simulink model "Grid_Forming_Converters_Microgrid_Github"  (R2020b)
settings: Solver=VariableStepAuto  StartTime=0.0  StopTime=1  RelTol=1e-3
values from neighbouring files (symbols this model uses):
  C_fi_1DG = 50*10^-6    (= 5e-05)    [Script_Primary_Secondary_Controller_GITHUB.m]
  C_fi_2DG = 50*10^-6    (= 5e-05)    [Script_Primary_Secondary_Controller_GITHUB.m]
  C_fi_3DG = 50*10^-6    (= 5e-05)    [Script_Primary_Secondary_Controller_GITHUB.m]
  C_fi_4DG = 50*10^-6    (= 5e-05)    [Script_Primary_Secondary_Controller_GITHUB.m]
  Kff_i_1DG = 0.75    [Script_Primary_Secondary_Controller_GITHUB.m]
  Kff_i_2DG = 0.75    [Script_Primary_Secondary_Controller_GITHUB.m]
  Kff_i_3DG = 0.75    [Script_Primary_Secondary_Controller_GITHUB.m]
  Kff_i_4DG = 0.75    [Script_Primary_Secondary_Controller_GITHUB.m]
  ki = 142500    [Script_Primary_Secondary_Controller_GITHUB.m]
  Kii_1DG = 20000    [Script_Primary_Secondary_Controller_GITHUB.m]
  Kii_2DG = 20000    [Script_Primary_Secondary_Controller_GITHUB.m]
  Kii_3DG = 16000    [Script_Primary_Secondary_Controller_GITHUB.m]
  Kii_4DG = 16000    [Script_Primary_Secondary_Controller_GITHUB.m]
  Kiv_1DG = 420    [Script_Primary_Secondary_Controller_GITHUB.m]
  Kiv_2DG = 420    [Script_Primary_Secondary_Controller_GITHUB.m]
  Kiv_3DG = 390    [Script_Primary_Secondary_Controller_GITHUB.m]
  Kiv_4DG = 390    [Script_Primary_Secondary_Controller_GITHUB.m]
  kp = 285    [Script_Primary_Secondary_Controller_GITHUB.m]
  Kpi_1DG = 15    [Script_Primary_Secondary_Controller_GITHUB.m]
  Kpi_2DG = 15    [Script_Primary_Secondary_Controller_GITHUB.m]
  Kpi_3DG = 10.5    [Script_Primary_Secondary_Controller_GITHUB.m]
  Kpi_4DG = 10.5    [Script_Primary_Secondary_Controller_GITHUB.m]
  Kpv_1DG = 0.1    [Script_Primary_Secondary_Controller_GITHUB.m]
  Kpv_2DG = 0.1    [Script_Primary_Secondary_Controller_GITHUB.m]
  Kpv_3DG = 0.05    [Script_Primary_Secondary_Controller_GITHUB.m]
  Kpv_4DG = 0.05    [Script_Primary_Secondary_Controller_GITHUB.m]
  L_ci_1DG = 0.35*10^-3    (= 0.00035)    [Script_Primary_Secondary_Controller_GITHUB.m]
  L_ci_2DG = 0.35*10^-3    (= 0.00035)    [Script_Primary_Secondary_Controller_GITHUB.m]
  L_fi_1DG = 1.35*10^-3    (= 0.00135)    [Script_Primary_Secondary_Controller_GITHUB.m]
  L_fi_2DG = 1.35*10^-3    (= 0.00135)    [Script_Primary_Secondary_Controller_GITHUB.m]
  L_fi_3DG = 1.35*10^-3    (= 0.00135)    [Script_Primary_Secondary_Controller_GITHUB.m]
  L_fi_4DG = 1.35*10^-3    (= 0.00135)    [Script_Primary_Secondary_Controller_GITHUB.m]
  L_line_1 = 318*10^-6    (= 0.000318)    [Script_Primary_Secondary_Controller_GITHUB.m]
  L_line_2 = 1847*10^-6    (= 0.001847)    [Script_Primary_Secondary_Controller_GITHUB.m]
  L_line_3 = 318*10^-6    (= 0.000318)    [Script_Primary_Secondary_Controller_GITHUB.m]
  L_load_1 = (X_load_1)/(2*pi*f)    (= 0.0477464829276)    [Script_Primary_Secondary_Controller_GITHUB.m]
  L_load_2 = (X_load_2)/(2*pi*f)    (= 0.0318309886184)    [Script_Primary_Secondary_Controller_GITHUB.m]
  L_load_3 = (X_load_3)/(2*pi*f)    (= 0.0318309886184)    [Script_Primary_Secondary_Controller_GITHUB.m]
  L_load_4 = (X_load_4)/(2*pi*f)    (= 0.0477464829276)    [Script_Primary_Secondary_Controller_GITHUB.m]
  m_P_1DG = 9.4*10^-5    (= 9.4e-05)    [Script_Primary_Secondary_Controller_GITHUB.m]
  m_P_2DG = 9.4*10^-5    (= 9.4e-05)    [Script_Primary_Secondary_Controller_GITHUB.m]
  m_P_3DG = 12.5*10^-5    (= 0.000125)    [Script_Primary_Secondary_Controller_GITHUB.m]
  m_P_4DG = 12.5*10^-5    (= 0.000125)    [Script_Primary_Secondary_Controller_GITHUB.m]
  n_Q_1DG = 1.3*10^-3    (= 0.0013)    [Script_Primary_Secondary_Controller_GITHUB.m]
  n_Q_2DG = 1.3*10^-3    (= 0.0013)    [Script_Primary_Secondary_Controller_GITHUB.m]
  n_Q_3DG = 1.5*10^-3    (= 0.0015)    [Script_Primary_Secondary_Controller_GITHUB.m]
  n_Q_4DG = 1.5*10^-3    (= 0.0015)    [Script_Primary_Secondary_Controller_GITHUB.m]
  R_ci_1DG = 0.03    [Script_Primary_Secondary_Controller_GITHUB.m]
  R_ci_2DG = 0.03    [Script_Primary_Secondary_Controller_GITHUB.m]
  R_fi_1DG = 0.1    [Script_Primary_Secondary_Controller_GITHUB.m]
  R_fi_2DG = 0.1    [Script_Primary_Secondary_Controller_GITHUB.m]
  R_fi_3DG = 0.1    [Script_Primary_Secondary_Controller_GITHUB.m]
  R_line_1 = 0.23    [Script_Primary_Secondary_Controller_GITHUB.m]
  R_line_2 = 0.35    [Script_Primary_Secondary_Controller_GITHUB.m]
  R_line_3 = 0.23    [Script_Primary_Secondary_Controller_GITHUB.m]
  R_load_1 = 30    [Script_Primary_Secondary_Controller_GITHUB.m]
  R_load_2 = 20    [Script_Primary_Secondary_Controller_GITHUB.m]
  R_load_3 = 25    [Script_Primary_Secondary_Controller_GITHUB.m]
  R_load_4 = 25    [Script_Primary_Secondary_Controller_GITHUB.m]
  Ts_1DG = 2e-6    (= 2e-06)    [Script_Primary_Secondary_Controller_GITHUB.m]
  w_base_1DG = 2*pi*f_1DG    (= 314.159265359)    [Script_Primary_Secondary_Controller_GITHUB.m]
  w_base_2DG = 2*pi*f_2DG    (= 314.159265359)    [Script_Primary_Secondary_Controller_GITHUB.m]
  w_base_3DG = 2*pi*f_3DG    (= 314.159265359)    [Script_Primary_Secondary_Controller_GITHUB.m]
  w_base_4DG = 2*pi*f_4DG    (= 314.159265359)    [Script_Primary_Secondary_Controller_GITHUB.m]
  wci_1DG = 31.41    [Script_Primary_Secondary_Controller_GITHUB.m]
  wci_2DG = 31.41    [Script_Primary_Secondary_Controller_GITHUB.m]
  wci_3DG = 31.41    [Script_Primary_Secondary_Controller_GITHUB.m]
  wci_4DG = 31.41    [Script_Primary_Secondary_Controller_GITHUB.m]
undefined symbols (not defined in the file or in its folder): L_i_1DG
libraries: powerlib x140, powerlib_meascontrol x68, pid_lib x20
(part 5 of 6)

== system Grid_Forming_Converters_Microgrid_Github/DG 3 VCVSI /Primary Controller DG 3/Current Loop Control 3 DG ==
  note: Vs_0*
  note: Vs_q*
  note: Vs_d*
  i_s_ref_dq0_3DG : Inport
  i_s_dq0_3DG : Inport  Port=2
  w_base_3DG : Inport  Port=3
  Constant : Constant  Value=0
  Demux : Demux  Outputs=2
  Demux2 : Demux  Outputs=2
  Gain : Gain  Gain=L_fi_3DG
  Mux : Mux  Inputs=3
  PID Controller : pid_lib/PID Controller  Controller=PI  Form=Parallel  TimeDomain=Continuous-time  UseExternalTs=off  SampleTime=-1  IntegratorMethod=Forward Euler  FilterMethod=Forward Euler  ControllerParametersSource=internal  P=Kpi_3DG  I=Kii_3DG  D=0  UseFilter=on  N=100  TunerSelectOption=Transfer Function Based (PID Tuner App)  InitialConditionSource=internal  InitialConditionForIntegrator=0  InitialConditionForFilter=0  DifferentiatorICPrevScaledInput=0  ExternalReset=none  TrackingMode=off  Kt=1  LimitOutput=off  SatLimitsSource=internal  UpperSaturationLimit=inf  LowerSaturationLimit=-inf  LinearizeAsGain=on  AntiWindupMode=none  Kb=1  POutMin=[]  POutMax=[]  IOutMin=[]  IOutMax=[]  DOutMin=[]  DOutMax=[]  NOutMin=[]  NOutMax=[]  SumOutMin=[]  SumOutMax=[]  SaturationOutMin=[]  SaturationOutMax=[]  PParamMin=[]  PParamMax=[]  IParamMin=[]  IParamMax=[]  DParamMin=[]  DParamMax=[]  NParamMin=[]  NParamMax=[]  KbParamMin=[]  KbParamMax=[]  KtParamMin=[]  KtParamMax=[]  KbOutMin=[]  KbOutMax=[]  KtOutMin=[]  KtOutMax=[]  IntegratorOutMin=[]  IntegratorOutMax=[]  FilterOutMin=[]  FilterOutMax=[]  SumI1OutMin=[]  SumI1OutMax=[]  SumI2OutMin=[]  SumI2OutMax=[]  SumI3OutMin=[]  SumI3OutMax=[]  SumI4OutMin=[]  SumI4OutMax=[]  SumDOutMin=[]  SumDOutMax=[]  DifferentiatorOutMin=[]  DifferentiatorOutMax=[]  FilterDiffOutCoefMin=[]  FilterDiffOutCoefMax=[]  ReciprocalOutMin=[]  ReciprocalOutMax=[]  SumDenOutMin=[]  SumDenOutMax=[]  SumNumOutMin=[]  SumNumOutMax=[]  DivideOutMin=[]  DivideOutMax=[]  UdiffTsProdOutMin=[]  UdiffTsProdOutMax=[]  NTsProdOutMin=[]  NTsProdOutMax=[]  UintegralTsProdOutMin=[]  UintegralTsProdOutMax=[]  UngainTsProdOutMin=[]  UngainTsProdOutMax=[]  IntegratorContinuousStateAttributes=''  IntegratorStateMustResolveToSignalObject=off  IntegratorRTWStateStorageClass=Auto  FilterContinuousStateAttributes=''  FilterStateMustResolveToSignalObject=off  FilterRTWStateStorageClass=Auto  ParallelPVariant=InternalParameters  IdealPVariant=Disabled  IVariant=InternalParameters  DVariant=Disabled  IntegratorVariant=Continuous  SatVariant=Disabled  AWVariant=Passthrough  PCopyVariant=Disabled  TRVariant=Disabled  FdbkBlocksVariant=Forward  IdealPFdbkVariant=Disabled  SatFdbkVariant=Disabled  DerivativeFilterVariant=Disabled  NVariant=Disabled  NCopyVariant=Disabled_SignalSpec  FilterICVariant=Disabled  IntegratorICVariant=InternalICs  ExternalResetVariant=Disabled  TRSumVariant=Passthrough  SumFdbkVariant=Disabled  SumVariant=Sum_PI  TsampFilterVariant=InternalTs  TsampNgainVariant=Passthrough  TsampIntegralVariant=Passthrough  ExternalSaturationOutDataTypeStr=Inherit: Same as second input
  PID Controller1 : pid_lib/PID Controller  Controller=PI  Form=Parallel  TimeDomain=Continuous-time  UseExternalTs=off  SampleTime=-1  IntegratorMethod=Forward Euler  FilterMethod=Forward Euler  ControllerParametersSource=internal  P=Kpi_3DG  I=Kii_3DG  D=0  UseFilter=on  N=100  TunerSelectOption=Transfer Function Based (PID Tuner App)  InitialConditionSource=internal  InitialConditionForIntegrator=0  InitialConditionForFilter=0  DifferentiatorICPrevScaledInput=0  ExternalReset=none  TrackingMode=off  Kt=1  LimitOutput=off  SatLimitsSource=internal  UpperSaturationLimit=inf  LowerSaturationLimit=-inf  LinearizeAsGain=on  AntiWindupMode=none  Kb=1  POutMin=[]  POutMax=[]  IOutMin=[]  IOutMax=[]  DOutMin=[]  DOutMax=[]  NOutMin=[]  NOutMax=[]  SumOutMin=[]  SumOutMax=[]  SaturationOutMin=[]  SaturationOutMax=[]  PParamMin=[]  PParamMax=[]  IParamMin=[]  IParamMax=[]  DParamMin=[]  DParamMax=[]  NParamMin=[]  NParamMax=[]  KbParamMin=[]  KbParamMax=[]  KtParamMin=[]  KtParamMax=[]  KbOutMin=[]  KbOutMax=[]  KtOutMin=[]  KtOutMax=[]  IntegratorOutMin=[]  IntegratorOutMax=[]  FilterOutMin=[]  FilterOutMax=[]  SumI1OutMin=[]  SumI1OutMax=[]  SumI2OutMin=[]  SumI2OutMax=[]  SumI3OutMin=[]  SumI3OutMax=[]  SumI4OutMin=[]  SumI4OutMax=[]  SumDOutMin=[]  SumDOutMax=[]  DifferentiatorOutMin=[]  DifferentiatorOutMax=[]  FilterDiffOutCoefMin=[]  FilterDiffOutCoefMax=[]  ReciprocalOutMin=[]  ReciprocalOutMax=[]  SumDenOutMin=[]  SumDenOutMax=[]  SumNumOutMin=[]  SumNumOutMax=[]  DivideOutMin=[]  DivideOutMax=[]  UdiffTsProdOutMin=[]  UdiffTsProdOutMax=[]  NTsProdOutMin=[]  NTsProdOutMax=[]  UintegralTsProdOutMin=[]  UintegralTsProdOutMax=[]  UngainTsProdOutMin=[]  UngainTsProdOutMax=[]  IntegratorContinuousStateAttributes=''  IntegratorStateMustResolveToSignalObject=off  IntegratorRTWStateStorageClass=Auto  FilterContinuousStateAttributes=''  FilterStateMustResolveToSignalObject=off  FilterRTWStateStorageClass=Auto  ParallelPVariant=InternalParameters  IdealPVariant=Disabled  IVariant=InternalParameters  DVariant=Disabled  IntegratorVariant=Continuous  SatVariant=Disabled  AWVariant=Passthrough  PCopyVariant=Disabled  TRVariant=Disabled  FdbkBlocksVariant=Forward  IdealPFdbkVariant=Disabled  SatFdbkVariant=Disabled  DerivativeFilterVariant=Disabled  NVariant=Disabled  NCopyVariant=Disabled_SignalSpec  FilterICVariant=Disabled  IntegratorICVariant=InternalICs  ExternalResetVariant=Disabled  TRSumVariant=Passthrough  SumFdbkVariant=Disabled  SumVariant=Sum_PI  TsampFilterVariant=InternalTs  TsampNgainVariant=Passthrough  TsampIntegralVariant=Passthrough  ExternalSaturationOutDataTypeStr=Inherit: Same as second input
  Product : Product
  Product1 : Product
  Selector1 : Selector  InputPortWidth=3  IndexOptions=Index vector (dialog)  Indices=[1 2]  OutputSizes=1
  Selector3 : Selector  InputPortWidth=3  IndexOptions=Index vector (dialog)  Indices=[1 2]  OutputSizes=1
  Sum : Sum  Inputs=|+-
  Sum1 : Sum  Inputs=|+-
  Sum2 : Sum  Inputs=|+-
  Sum3 : Sum  Inputs=|++
  powergui : powerlib/powergui  Priority=1  SimulationMode=Discrete  SampleTime=2e-6  frequency=60  Iterations=50  frequencyindice=0  Pbase=100e6  ErrMax=1e-4  UnitsV=kV  UnitsW=MW  buscounter=0  FunctionMessages=off  echomessages=off  EnableUseOfTLC=off  CurrentSourceSwitches=off  DisableSnubberDevices=off  DisableRonSwitches=off  DisableVfSwitches=off  DisplayEquations=off  AutomaticDiscreteSolvers=off  SolverType=Tustin/Backward Euler (TBE)  Interpol=off  ExternalGateDelay=off  methode=off  Ts=100  x0status=blocks  SPID=on  SwTol=0  HookPort=off  NonlinearTolerance=1e-4  nMaxIteration=100  ContinueOnMaxIteration=off  RestoreLinks=warning  ResistiveCurrentMeasurement=off  Frange=[0:2:500]  Ylog=off  Xlog=on  ShowGrid=off  save=off  variable=ZData  structure=0  ZoomFFT=off  StartTime=0.0  cycles=1  DisplayStyle=1  fundamental=60  FreqAxis=off  MaxFrequency=1000  frequencyindicesteady=1  RmsSteady=1  display=off
  v_s_ref_dq0_3DG : Outport
  wires:
  i_s_ref_dq0_3DG/1 -> Selector1/1
  Selector1/1 -> Demux/1
  i_s_dq0_3DG/1 -> Selector3/1
  Selector3/1 -> Demux2/1
  Demux/1 -> Sum/1
  Demux2/1 -> Product1/2, Sum/2
  Sum/1 -> PID Controller/1
  PID Controller/1 -> Sum1/1
  w_base_3DG/1 -> Gain/1
  Gain/1 -> Product1/1, Product/1
  Demux2/2 -> Product/2, Sum2/2
  Product/1 -> Sum1/2
  Demux/2 -> Sum2/1
  Sum2/1 -> PID Controller1/1
  PID Controller1/1 -> Sum3/1
  Product1/1 -> Sum3/2
  Mux/1 -> v_s_ref_dq0_3DG/1
  Sum1/1 -> Mux/1
  Sum3/1 -> Mux/2
  Constant/1 -> Mux/3

== system Grid_Forming_Converters_Microgrid_Github/DG 3 VCVSI /Primary Controller DG 3/Droop Control Subsystem 3 DG ==
  Q_3DG : Inport
  P_3DG : Inport  Port=2
  w_n_3DG : Inport  Port=3
  V_n_3DG : Inport  Port=4
  Constant : Constant  Value=0
  Gain : Gain  Gain=m_P_3DG
  Gain1 : Gain  Gain=n_Q_3DG
  Gain2 : Gain  Gain=1/(2*pi)
  Mux : Mux  Inputs=3
  Sum : Sum  Inputs=|+-
  Sum1 : Sum  Inputs=|+-
  powergui : powerlib/powergui  Priority=1  SimulationMode=Discrete  SampleTime=2e-6  frequency=60  Iterations=50  frequencyindice=0  Pbase=100e6  ErrMax=1e-4  UnitsV=kV  UnitsW=MW  buscounter=0  FunctionMessages=off  echomessages=off  EnableUseOfTLC=off  CurrentSourceSwitches=off  DisableSnubberDevices=off  DisableRonSwitches=off  DisableVfSwitches=off  DisplayEquations=off  AutomaticDiscreteSolvers=off  SolverType=Tustin/Backward Euler (TBE)  Interpol=off  ExternalGateDelay=off  methode=off  Ts=100  x0status=blocks  SPID=on  SwTol=0  HookPort=off  NonlinearTolerance=1e-4  nMaxIteration=100  ContinueOnMaxIteration=off  RestoreLinks=warning  ResistiveCurrentMeasurement=off  Frange=[0:2:500]  Ylog=off  Xlog=on  ShowGrid=off  save=off  variable=ZData  structure=0  ZoomFFT=off  StartTime=0.0  cycles=1  DisplayStyle=1  fundamental=60  FreqAxis=off  MaxFrequency=1000  frequencyindicesteady=1  RmsSteady=1  display=off
  w_3DG : Outport
  frequency_3DG : Outport  Port=2
  v_ref_dq0_3DG : Outport  Port=3
  wires:
  P_3DG/1 -> Gain/1
  Q_3DG/1 -> Gain1/1
  w_n_3DG/1 -> Sum/1
  Gain/1 -> Sum/2
  V_n_3DG/1 -> Sum1/1
  Gain1/1 -> Sum1/2
  Sum/1 -> Gain2/1, w_3DG/1
  Sum1/1 -> [v_odi_star_3DG], Mux/1
  Mux/1 -> v_ref_dq0_3DG/1
  Constant/1 -> [v_oq_star_3DG], Mux/3, Mux/2
  Gain2/1 -> frequency_3DG/1

== system Grid_Forming_Converters_Microgrid_Github/DG 3 VCVSI /Primary Controller DG 3/Voltage Loop Control 3 DG ==
  note: Is_d*
  note: Is_q*
  v_ref_dq0_3DG : Inport
  v_dq0_3DG : Inport  Port=2
  i_dq0_3DG : Inport  Port=3
  w_base_3DG : Inport  Port=4
  Demux : Demux  Outputs=2
  Demux1 : Demux  Outputs=2
  Demux2 : Demux  Outputs=2
  Gain : Gain  Gain=C_fi_3DG
  Gain1 : Gain  Gain=Kff_i_3DG
  Gain2 : Gain  Gain=Kff_i_3DG
  Is_0* : Constant  Value=0
  Mux : Mux  Inputs=3
  PID Controller : pid_lib/PID Controller  Controller=PI  Form=Parallel  TimeDomain=Continuous-time  UseExternalTs=off  SampleTime=-1  IntegratorMethod=Forward Euler  FilterMethod=Forward Euler  ControllerParametersSource=internal  P=Kpv_3DG  I=Kiv_3DG  D=0  UseFilter=on  N=100  TunerSelectOption=Transfer Function Based (PID Tuner App)  InitialConditionSource=internal  InitialConditionForIntegrator=0  InitialConditionForFilter=0  DifferentiatorICPrevScaledInput=0  ExternalReset=none  TrackingMode=off  Kt=1  LimitOutput=off  SatLimitsSource=internal  UpperSaturationLimit=inf  LowerSaturationLimit=-inf  LinearizeAsGain=on  AntiWindupMode=none  Kb=1  POutMin=[]  POutMax=[]  IOutMin=[]  IOutMax=[]  DOutMin=[]  DOutMax=[]  NOutMin=[]  NOutMax=[]  SumOutMin=[]  SumOutMax=[]  SaturationOutMin=[]  SaturationOutMax=[]  PParamMin=[]  PParamMax=[]  IParamMin=[]  IParamMax=[]  DParamMin=[]  DParamMax=[]  NParamMin=[]  NParamMax=[]  KbParamMin=[]  KbParamMax=[]  KtParamMin=[]  KtParamMax=[]  KbOutMin=[]  KbOutMax=[]  KtOutMin=[]  KtOutMax=[]  IntegratorOutMin=[]  IntegratorOutMax=[]  FilterOutMin=[]  FilterOutMax=[]  SumI1OutMin=[]  SumI1OutMax=[]  SumI2OutMin=[]  SumI2OutMax=[]  SumI3OutMin=[]  SumI3OutMax=[]  SumI4OutMin=[]  SumI4OutMax=[]  SumDOutMin=[]  SumDOutMax=[]  DifferentiatorOutMin=[]  DifferentiatorOutMax=[]  FilterDiffOutCoefMin=[]  FilterDiffOutCoefMax=[]  ReciprocalOutMin=[]  ReciprocalOutMax=[]  SumDenOutMin=[]  SumDenOutMax=[]  SumNumOutMin=[]  SumNumOutMax=[]  DivideOutMin=[]  DivideOutMax=[]  UdiffTsProdOutMin=[]  UdiffTsProdOutMax=[]  NTsProdOutMin=[]  NTsProdOutMax=[]  UintegralTsProdOutMin=[]  UintegralTsProdOutMax=[]  UngainTsProdOutMin=[]  UngainTsProdOutMax=[]  IntegratorContinuousStateAttributes=''  IntegratorStateMustResolveToSignalObject=off  IntegratorRTWStateStorageClass=Auto  FilterContinuousStateAttributes=''  FilterStateMustResolveToSignalObject=off  FilterRTWStateStorageClass=Auto  ParallelPVariant=InternalParameters  IdealPVariant=Disabled  IVariant=InternalParameters  DVariant=Disabled  IntegratorVariant=Continuous  SatVariant=Disabled  AWVariant=Passthrough  PCopyVariant=Disabled  TRVariant=Disabled  FdbkBlocksVariant=Forward  IdealPFdbkVariant=Disabled  SatFdbkVariant=Disabled  DerivativeFilterVariant=Disabled  NVariant=Disabled  NCopyVariant=Disabled_SignalSpec  FilterICVariant=Disabled  IntegratorICVariant=InternalICs  ExternalResetVariant=Disabled  TRSumVariant=Passthrough  SumFdbkVariant=Disabled  SumVariant=Sum_PI  TsampFilterVariant=InternalTs  TsampNgainVariant=Passthrough  TsampIntegralVariant=Passthrough  ExternalSaturationOutDataTypeStr=Inherit: Same as second input
  PID Controller2 : pid_lib/PID Controller  Controller=PI  Form=Parallel  TimeDomain=Continuous-time  UseExternalTs=off  SampleTime=-1  IntegratorMethod=Forward Euler  FilterMethod=Forward Euler  ControllerParametersSource=internal  P=Kpv_3DG  I=Kiv_3DG  D=0  UseFilter=on  N=100  TunerSelectOption=Transfer Function Based (PID Tuner App)  InitialConditionSource=internal  InitialConditionForIntegrator=0  InitialConditionForFilter=0  DifferentiatorICPrevScaledInput=0  ExternalReset=none  TrackingMode=off  Kt=1  LimitOutput=off  SatLimitsSource=internal  UpperSaturationLimit=inf  LowerSaturationLimit=-inf  LinearizeAsGain=on  AntiWindupMode=none  Kb=1  POutMin=[]  POutMax=[]  IOutMin=[]  IOutMax=[]  DOutMin=[]  DOutMax=[]  NOutMin=[]  NOutMax=[]  SumOutMin=[]  SumOutMax=[]  SaturationOutMin=[]  SaturationOutMax=[]  PParamMin=[]  PParamMax=[]  IParamMin=[]  IParamMax=[]  DParamMin=[]  DParamMax=[]  NParamMin=[]  NParamMax=[]  KbParamMin=[]  KbParamMax=[]  KtParamMin=[]  KtParamMax=[]  KbOutMin=[]  KbOutMax=[]  KtOutMin=[]  KtOutMax=[]  IntegratorOutMin=[]  IntegratorOutMax=[]  FilterOutMin=[]  FilterOutMax=[]  SumI1OutMin=[]  SumI1OutMax=[]  SumI2OutMin=[]  SumI2OutMax=[]  SumI3OutMin=[]  SumI3OutMax=[]  SumI4OutMin=[]  SumI4OutMax=[]  SumDOutMin=[]  SumDOutMax=[]  DifferentiatorOutMin=[]  DifferentiatorOutMax=[]  FilterDiffOutCoefMin=[]  FilterDiffOutCoefMax=[]  ReciprocalOutMin=[]  ReciprocalOutMax=[]  SumDenOutMin=[]  SumDenOutMax=[]  SumNumOutMin=[]  SumNumOutMax=[]  DivideOutMin=[]  DivideOutMax=[]  UdiffTsProdOutMin=[]  UdiffTsProdOutMax=[]  NTsProdOutMin=[]  NTsProdOutMax=[]  UintegralTsProdOutMin=[]  UintegralTsProdOutMax=[]  UngainTsProdOutMin=[]  UngainTsProdOutMax=[]  IntegratorContinuousStateAttributes=''  IntegratorStateMustResolveToSignalObject=off  IntegratorRTWStateStorageClass=Auto  FilterContinuousStateAttributes=''  FilterStateMustResolveToSignalObject=off  FilterRTWStateStorageClass=Auto  ParallelPVariant=InternalParameters  IdealPVariant=Disabled  IVariant=InternalParameters  DVariant=Disabled  IntegratorVariant=Continuous  SatVariant=Disabled  AWVariant=Passthrough  PCopyVariant=Disabled  TRVariant=Disabled  FdbkBlocksVariant=Forward  IdealPFdbkVariant=Disabled  SatFdbkVariant=Disabled  DerivativeFilterVariant=Disabled  NVariant=Disabled  NCopyVariant=Disabled_SignalSpec  FilterICVariant=Disabled  IntegratorICVariant=InternalICs  ExternalResetVariant=Disabled  TRSumVariant=Passthrough  SumFdbkVariant=Disabled  SumVariant=Sum_PI  TsampFilterVariant=InternalTs  TsampNgainVariant=Passthrough  TsampIntegralVariant=Passthrough  ExternalSaturationOutDataTypeStr=Inherit: Same as second input
  Product : Product
  Product1 : Product
  Scope1 : Scope
  Scope8 : Scope
  Selector1 : Selector  InputPortWidth=3  IndexOptions=Index vector (dialog)  Indices=[1 2]  OutputSizes=1
  Selector2 : Selector  InputPortWidth=3  IndexOptions=Index vector (dialog)  Indices=[1 2]  OutputSizes=1
  Selector3 : Selector  InputPortWidth=3  IndexOptions=Index vector (dialog)  Indices=[1 2]  OutputSizes=1
  Sum : Sum  Inputs=|+-
  Sum1 : Sum  Inputs=|+-
  Sum2 : Sum  Inputs=|+-
  Sum3 : Sum  Inputs=|++
  Sum4 : Sum  Inputs=|++
  Sum5 : Sum  Inputs=|++
  powergui : powerlib/powergui  Priority=1  SimulationMode=Discrete  SampleTime=2e-6  frequency=60  Iterations=50  frequencyindice=0  Pbase=100e6  ErrMax=1e-4  UnitsV=kV  UnitsW=MW  buscounter=0  FunctionMessages=off  echomessages=off  EnableUseOfTLC=off  CurrentSourceSwitches=off  DisableSnubberDevices=off  DisableRonSwitches=off  DisableVfSwitches=off  DisplayEquations=off  AutomaticDiscreteSolvers=off  SolverType=Tustin/Backward Euler (TBE)  Interpol=off  ExternalGateDelay=off  methode=off  Ts=100  x0status=blocks  SPID=on  SwTol=0  HookPort=off  NonlinearTolerance=1e-4  nMaxIteration=100  ContinueOnMaxIteration=off  RestoreLinks=warning  ResistiveCurrentMeasurement=off  Frange=[0:2:500]  Ylog=off  Xlog=on  ShowGrid=off  save=off  variable=ZData  structure=0  ZoomFFT=off  StartTime=0.0  cycles=1  DisplayStyle=1  fundamental=60  FreqAxis=off  MaxFrequency=1000  frequencyindicesteady=1  RmsSteady=1  display=off
  i_s_ref_dq0_3DG : Outport
  wires:
  v_ref_dq0_3DG/1 -> Selector1/1
  Selector1/1 -> Demux/1
  Demux/1 -> Sum/1  "Eg_d*"
  v_dq0_3DG/1 -> Selector2/1
  Selector2/1 -> Demux1/1
  Demux1/1 -> Scope8/1, Product1/1, Sum/2  "Eg_d"
  Demux/2 -> Sum1/1  "Eg_q*"
  Demux1/2 -> Sum1/2, Scope1/1, Product/2  "Eg_q"
  Sum1/1 -> PID Controller/1
  PID Controller/1 -> Sum3/1
  w_base_3DG/1 -> Gain/1
  Gain/1 -> Product1/2, Product/1
  Product/1 -> Sum2/2
  Sum2/1 -> Sum4/1
  i_dq0_3DG/1 -> Selector3/1
  Selector3/1 -> Demux2/1
  Product1/1 -> Sum3/2
  Sum3/1 -> Sum5/1
  Gain1/1 -> Sum4/2
  Demux2/1 -> Gain1/1  "Eg_d"
  Demux2/2 -> Gain2/1  "Eg_q"
  Gain2/1 -> Sum5/2
  Sum4/1 -> [i_1d_star_3DG], Mux/1
  Sum5/1 -> [i_1q_star_3DG], Mux/2
  Is_0*/1 -> Mux/3
  Mux/1 -> i_s_ref_dq0_3DG/1
  Sum/1 -> PID Controller2/1
  PID Controller2/1 -> Sum2/1

== system Grid_Forming_Converters_Microgrid_Github/DG 3 VCVSI /Primary Controller DG 3/convertion block dq to abc frame 3 DG ==
  v_s_ref_dq0_3DG : Inport
  alpha_3DG : Inport  Port=2
  Display23 : Display
  Scope48 : Scope
  dq0 to abc : powerlib_meascontrol/Transformations/dq0 to abc  Alignment=90 degrees behind phase A axis
  powergui : powerlib/powergui  Priority=1  SimulationMode=Discrete  SampleTime=2e-6  frequency=60  Iterations=50  frequencyindice=0  Pbase=100e6  ErrMax=1e-4  UnitsV=kV  UnitsW=MW  buscounter=0  FunctionMessages=off  echomessages=off  EnableUseOfTLC=off  CurrentSourceSwitches=off  DisableSnubberDevices=off  DisableRonSwitches=off  DisableVfSwitches=off  DisplayEquations=off  AutomaticDiscreteSolvers=off  SolverType=Tustin/Backward Euler (TBE)  Interpol=off  ExternalGateDelay=off  methode=off  Ts=100  x0status=blocks  SPID=on  SwTol=0  HookPort=off  NonlinearTolerance=1e-4  nMaxIteration=100  ContinueOnMaxIteration=off  RestoreLinks=warning  ResistiveCurrentMeasurement=off  Frange=[0:2:500]  Ylog=off  Xlog=on  ShowGrid=off  save=off  variable=ZData  structure=0  ZoomFFT=off  StartTime=0.0  cycles=1  DisplayStyle=1  fundamental=60  FreqAxis=off  MaxFrequency=1000  frequencyindicesteady=1  RmsSteady=1  display=off
  voltage_abc_DG3 : Outport
  wires:
  dq0 to abc/1 -> voltage_abc_DG3/1
  v_s_ref_dq0_3DG/1 -> Scope48/1, dq0 to abc/1, Display23/1
  alpha_3DG/1 -> dq0 to abc/2

== system Grid_Forming_Converters_Microgrid_Github/DG 4 VCVSI /Conversion and Measurement Block from abc to dq0 frame/Measurement block ==
  v_dq0_4DG : Inport
  i_s_dq0_4DG : Inport  Port=2
  i_dq0_4DG : Inport  Port=3
  v_bus_dq0_4DG : Inport  Port=4
  v_s_dq0_4DG : Inport  Port=5
  Demux{1..5} (5 alike) : Demux  Outputs=3
  Display1 : Display
  Display2 : Display
  Display25 : Display
  Low Pass Filter d : Subsystem
  Low Pass Filter q : Subsystem
  Math Function : Math  Operator=square  SaturateOnIntegerOverflow=on
  Math Function1 : Math  Operator=square  SaturateOnIntegerOverflow=on
  Scope1 : Scope
  Scope2 : Scope
  Scope33 : Scope
  Sqrt2 : Sqrt  SaturateOnIntegerOverflow=on
  Sum2 : Sum  Inputs=|++
  Terminator{1..5} (5 alike) : Terminator
  powergui : powerlib/powergui  Priority=1  SimulationMode=Discrete  SampleTime=2e-6  frequency=60  Iterations=50  frequencyindice=0  Pbase=100e6  ErrMax=1e-4  UnitsV=kV  UnitsW=MW  buscounter=0  FunctionMessages=off  echomessages=off  EnableUseOfTLC=off  CurrentSourceSwitches=off  DisableSnubberDevices=off  DisableRonSwitches=off  DisableVfSwitches=off  DisplayEquations=off  AutomaticDiscreteSolvers=off  SolverType=Tustin/Backward Euler (TBE)  Interpol=off  ExternalGateDelay=off  methode=off  Ts=100  x0status=blocks  SPID=on  SwTol=0  HookPort=off  NonlinearTolerance=1e-4  nMaxIteration=100  ContinueOnMaxIteration=off  RestoreLinks=warning  ResistiveCurrentMeasurement=off  Frange=[0:2:500]  Ylog=off  Xlog=on  ShowGrid=off  save=off  variable=ZData  structure=0  ZoomFFT=off  StartTime=0.0  cycles=1  DisplayStyle=1  fundamental=60  FreqAxis=off  MaxFrequency=1000  frequencyindicesteady=1  RmsSteady=1  display=off
  vo_mag_4DG : Outport
  v_od_4DG : Outport  Port=2
  v_oq_4DG : Outport  Port=3
  i_1d_4DG : Outport  Port=4
  i_1q_4DG : Outport  Port=5
  i_od_4DG : Outport  Port=6
  i_oq_4DG : Outport  Port=7
  v_bd_4DG : Outport  Port=8
  v_bq_4DG : Outport  Port=9
  v_id_4DG : Outport  Port=10
  v_iq_4DG : Outport  Port=11
  wires:
  Sum2/1 -> Sqrt2/1
  i_dq0_4DG/1 -> Demux3/1
  Sqrt2/1 -> Display25/1, Scope33/1, vo_mag_4DG/1
  Demux1/3 -> Terminator1/1  "0"
  Demux1/2 -> i_1q_4DG/1  "q"
  Math Function/1 -> Sum2/1
  Demux3/3 -> Terminator2/1  "0"
  Demux2/3 -> Terminator4/1  "0"
  Math Function1/1 -> Sum2/2
  i_s_dq0_4DG/1 -> Demux1/1
  Demux3/2 -> i_oq_4DG/1  "q"
  Demux3/1 -> i_od_4DG/1  "d"
  Demux1/1 -> i_1d_4DG/1  "d"
  v_dq0_4DG/1 -> Demux2/1
  Demux2/1 -> Low Pass Filter d/1(In1)  "d"
  Low Pass Filter d/1(Out1) -> Display1/1, Scope1/1, v_od_4DG/1, Math Function/1
  Demux2/2 -> Low Pass Filter q/1(In1)  "q"
  Low Pass Filter q/1(Out1) -> Scope2/1, Display2/1, v_oq_4DG/1, Math Function1/1
  Demux4/3 -> Terminator3/1  "0"
  Demux5/2 -> v_iq_4DG/1  "q"
  v_s_dq0_4DG/1 -> Demux5/1
  Demux4/1 -> v_bd_4DG/1  "d"
  Demux5/1 -> v_id_4DG/1  "d"
  v_bus_dq0_4DG/1 -> Demux4/1
  Demux5/3 -> Terminator5/1  "0"
  Demux4/2 -> v_bq_4DG/1  "q"

== system Grid_Forming_Converters_Microgrid_Github/DG 4 VCVSI /Conversion and Measurement Block from abc to dq0 frame/abc to dq0 frame ==
  alpha_4DG : Inport
  i_abc_4DG : Inport  Port=2
  i_s_abc_4DG : Inport  Port=3
  v_abc_4DG : Inport  Port=4
  v_bus_abc_4DG : Inport  Port=5
  v_s_abc_4DG : Inport  Port=6
  Alpha-Beta-Zero to dq0 {1..5} (5 alike) : powerlib_meascontrol/Transformations/Alpha-Beta-Zero to dq0  Alignment=90 degrees behind phase A axis
  abc to Alpha-Beta-Zero{1..5} (5 alike) : powerlib_meascontrol/Transformations/abc to Alpha-Beta-Zero
  powergui : powerlib/powergui  Priority=1  SimulationMode=Discrete  SampleTime=2e-6  frequency=60  Iterations=50  frequencyindice=0  Pbase=100e6  ErrMax=1e-4  UnitsV=kV  UnitsW=MW  buscounter=0  FunctionMessages=off  echomessages=off  EnableUseOfTLC=off  CurrentSourceSwitches=off  DisableSnubberDevices=off  DisableRonSwitches=off  DisableVfSwitches=off  DisplayEquations=off  AutomaticDiscreteSolvers=off  SolverType=Tustin/Backward Euler (TBE)  Interpol=off  ExternalGateDelay=off  methode=off  Ts=100  x0status=blocks  SPID=on  SwTol=0  HookPort=off  NonlinearTolerance=1e-4  nMaxIteration=100  ContinueOnMaxIteration=off  RestoreLinks=warning  ResistiveCurrentMeasurement=off  Frange=[0:2:500]  Ylog=off  Xlog=on  ShowGrid=off  save=off  variable=ZData  structure=0  ZoomFFT=off  StartTime=0.0  cycles=1  DisplayStyle=1  fundamental=60  FreqAxis=off  MaxFrequency=1000  frequencyindicesteady=1  RmsSteady=1  display=off
  i_dq0_4DG : Outport
  i_s_dq0_4DG : Outport  Port=2
  v_dq0_4DG : Outport  Port=3
  v_bus_dq0_4DG : Outport  Port=4
  v_s_dq0_4DG : Outport  Port=5
  wires:
  i_abc_4DG/1 -> abc to Alpha-Beta-Zero1/1
  abc to Alpha-Beta-Zero1/1 -> Alpha-Beta-Zero to dq0 2/1
  Alpha-Beta-Zero to dq0 2/1 -> i_dq0_4DG/1
  i_s_abc_4DG/1 -> abc to Alpha-Beta-Zero2/1
  abc to Alpha-Beta-Zero2/1 -> Alpha-Beta-Zero to dq0 1/1
  Alpha-Beta-Zero to dq0 1/1 -> i_s_dq0_4DG/1
  v_abc_4DG/1 -> abc to Alpha-Beta-Zero4/1
  abc to Alpha-Beta-Zero4/1 -> Alpha-Beta-Zero to dq0 4/1
  Alpha-Beta-Zero to dq0 4/1 -> v_dq0_4DG/1
  alpha_4DG/1 -> Alpha-Beta-Zero to dq0 4/2, Alpha-Beta-Zero to dq0 3/2, Alpha-Beta-Zero to dq0 5/2, Alpha-Beta-Zero to dq0 1/2, Alpha-Beta-Zero to dq0 2/2
  Alpha-Beta-Zero to dq0 3/1 -> v_bus_dq0_4DG/1
  v_bus_abc_4DG/1 -> abc to Alpha-Beta-Zero3/1
  abc to Alpha-Beta-Zero3/1 -> Alpha-Beta-Zero to dq0 3/1
  Alpha-Beta-Zero to dq0 5/1 -> v_s_dq0_4DG/1
  v_s_abc_4DG/1 -> abc to Alpha-Beta-Zero5/1
  abc to Alpha-Beta-Zero5/1 -> Alpha-Beta-Zero to dq0 5/1

== system Grid_Forming_Converters_Microgrid_Github/DG 4 VCVSI /Conversion and Measurement Block from abc to dq0 frame/alpha_calculator_4DG ==
  v_oq_4DG : Inport
  Constant : Constant  Value=0
  Integrator : Integrator
  PID Controller : pid_lib/PID Controller  Controller=PI  Form=Parallel  TimeDomain=Continuous-time  UseExternalTs=off  SampleTime=-1  IntegratorMethod=Forward Euler  FilterMethod=Forward Euler  ControllerParametersSource=internal  P=kp  I=ki  D=0  UseFilter=on  N=100  TunerSelectOption=Transfer Function Based (PID Tuner App)  InitialConditionSource=internal  InitialConditionForIntegrator=0  InitialConditionForFilter=0  DifferentiatorICPrevScaledInput=0  ExternalReset=none  TrackingMode=off  Kt=1  LimitOutput=off  SatLimitsSource=internal  UpperSaturationLimit=inf  LowerSaturationLimit=-inf  LinearizeAsGain=on  AntiWindupMode=none  Kb=1  POutMin=[]  POutMax=[]  IOutMin=[]  IOutMax=[]  DOutMin=[]  DOutMax=[]  NOutMin=[]  NOutMax=[]  SumOutMin=[]  SumOutMax=[]  SaturationOutMin=[]  SaturationOutMax=[]  PParamMin=[]  PParamMax=[]  IParamMin=[]  IParamMax=[]  DParamMin=[]  DParamMax=[]  NParamMin=[]  NParamMax=[]  KbParamMin=[]  KbParamMax=[]  KtParamMin=[]  KtParamMax=[]  KbOutMin=[]  KbOutMax=[]  KtOutMin=[]  KtOutMax=[]  IntegratorOutMin=[]  IntegratorOutMax=[]  FilterOutMin=[]  FilterOutMax=[]  SumI1OutMin=[]  SumI1OutMax=[]  SumI2OutMin=[]  SumI2OutMax=[]  SumI3OutMin=[]  SumI3OutMax=[]  SumI4OutMin=[]  SumI4OutMax=[]  SumDOutMin=[]  SumDOutMax=[]  DifferentiatorOutMin=[]  DifferentiatorOutMax=[]  FilterDiffOutCoefMin=[]  FilterDiffOutCoefMax=[]  ReciprocalOutMin=[]  ReciprocalOutMax=[]  SumDenOutMin=[]  SumDenOutMax=[]  SumNumOutMin=[]  SumNumOutMax=[]  DivideOutMin=[]  DivideOutMax=[]  UdiffTsProdOutMin=[]  UdiffTsProdOutMax=[]  NTsProdOutMin=[]  NTsProdOutMax=[]  UintegralTsProdOutMin=[]  UintegralTsProdOutMax=[]  UngainTsProdOutMin=[]  UngainTsProdOutMax=[]  IntegratorContinuousStateAttributes=''  IntegratorStateMustResolveToSignalObject=off  IntegratorRTWStateStorageClass=Auto  FilterContinuousStateAttributes=''  FilterStateMustResolveToSignalObject=off  FilterRTWStateStorageClass=Auto  ParallelPVariant=InternalParameters  IdealPVariant=Disabled  IVariant=InternalParameters  DVariant=Disabled  IntegratorVariant=Continuous  SatVariant=Disabled  AWVariant=Passthrough  PCopyVariant=Disabled  TRVariant=Disabled  FdbkBlocksVariant=Forward  IdealPFdbkVariant=Disabled  SatFdbkVariant=Disabled  DerivativeFilterVariant=Disabled  NVariant=Disabled  NCopyVariant=Disabled_SignalSpec  FilterICVariant=Disabled  IntegratorICVariant=InternalICs  ExternalResetVariant=Disabled  TRSumVariant=Passthrough  SumFdbkVariant=Disabled  SumVariant=Sum_PI  TsampFilterVariant=InternalTs  TsampNgainVariant=Passthrough  TsampIntegralVariant=Passthrough  ExternalSaturationOutDataTypeStr=Inherit: Same as second input
  Sum : Sum  Inputs=|+-
  powergui : powerlib/powergui  Priority=1  SimulationMode=Discrete  SampleTime=2e-6  frequency=60  Iterations=50  frequencyindice=0  Pbase=100e6  ErrMax=1e-4  UnitsV=kV  UnitsW=MW  buscounter=0  FunctionMessages=off  echomessages=off  EnableUseOfTLC=off  CurrentSourceSwitches=off  DisableSnubberDevices=off  DisableRonSwitches=off  DisableVfSwitches=off  DisplayEquations=off  AutomaticDiscreteSolvers=off  SolverType=Tustin/Backward Euler (TBE)  Interpol=off  ExternalGateDelay=off  methode=off  Ts=100  x0status=blocks  SPID=on  SwTol=0  HookPort=off  NonlinearTolerance=1e-4  nMaxIteration=100  ContinueOnMaxIteration=off  RestoreLinks=warning  ResistiveCurrentMeasurement=off  Frange=[0:2:500]  Ylog=off  Xlog=on  ShowGrid=off  save=off  variable=ZData  structure=0  ZoomFFT=off  StartTime=0.0  cycles=1  DisplayStyle=1  fundamental=60  FreqAxis=off  MaxFrequency=1000  frequencyindicesteady=1  RmsSteady=1  display=off
  alpha_4DG : Outport
  wires:
  v_oq_4DG/1 -> Sum/2
  Constant/1 -> Sum/1
  Sum/1 -> PID Controller/1
  PID Controller/1 -> Integrator/1
  Integrator/1 -> alpha_4DG/1

== system Grid_Forming_Converters_Microgrid_Github/DG 4 VCVSI /Primary Controller DG 4/Active and Reactive Power ==
  v_od_4DG : Inport
  i_od_4DG : Inport  Port=2
  v_oq_4DG : Inport  Port=3
  i_oq_4DG : Inport  Port=4
  Product{,1..3} (4 alike) : Product
  Sum : Sum  Inputs=|++
  Sum1 : Sum  Inputs=|+-
  Transfer Fcn : TransferFcn  Numerator=[wci_4DG]  Denominator=[1 wci_4DG]
  Transfer Fcn1 : TransferFcn  Numerator=[wci_4DG]  Denominator=[1 wci_4DG]
  powergui : powerlib/powergui  Priority=1  SimulationMode=Discrete  SampleTime=2e-6  frequency=60  Iterations=50  frequencyindice=0  Pbase=100e6  ErrMax=1e-4  UnitsV=kV  UnitsW=MW  buscounter=0  FunctionMessages=off  echomessages=off  EnableUseOfTLC=off  CurrentSourceSwitches=off  DisableSnubberDevices=off  DisableRonSwitches=off  DisableVfSwitches=off  DisplayEquations=off  AutomaticDiscreteSolvers=off  SolverType=Tustin/Backward Euler (TBE)  Interpol=off  ExternalGateDelay=off  methode=off  Ts=100  x0status=blocks  SPID=on  SwTol=0  HookPort=off  NonlinearTolerance=1e-4  nMaxIteration=100  ContinueOnMaxIteration=off  RestoreLinks=warning  ResistiveCurrentMeasurement=off  Frange=[0:2:500]  Ylog=off  Xlog=on  ShowGrid=off  save=off  variable=ZData  structure=0  ZoomFFT=off  StartTime=0.0  cycles=1  DisplayStyle=1  fundamental=60  FreqAxis=off  MaxFrequency=1000  frequencyindicesteady=1  RmsSteady=1  display=off
  P_4DG : Outport
  Q_4DG : Outport  Port=2
  wires:
  v_od_4DG/1 -> Product3/1, Product/1
  i_od_4DG/1 -> Product2/2, Product/2
  v_oq_4DG/1 -> Product2/1, Product1/1
  i_oq_4DG/1 -> Product3/2, Product1/2
  Product/1 -> Sum/1
  Product1/1 -> Sum/2
  Sum/1 -> [P_i_instant_4DG], Transfer Fcn/1
  Transfer Fcn/1 -> P_4DG/1
  Sum1/1 -> [Q_i_instant_4DG], Transfer Fcn1/1
  Transfer Fcn1/1 -> Q_4DG/1
  Product2/1 -> Sum1/1
  Product3/1 -> Sum1/2

== system Grid_Forming_Converters_Microgrid_Github/DG 4 VCVSI /Primary Controller DG 4/Current Loop Control 4 DG ==
  note: Vs_0*
  note: Vs_q*
  note: Vs_d*
  i_s_ref_dq0_4DG : Inport
  i_s_dq0_4DG : Inport  Port=2
  w_base_4DG : Inport  Port=3
  Constant : Constant  Value=0
  Demux : Demux  Outputs=2
  Demux2 : Demux  Outputs=2
  Gain : Gain  Gain=L_fi_4DG
  Mux : Mux  Inputs=3
  PID Controller : pid_lib/PID Controller  Controller=PI  Form=Parallel  TimeDomain=Continuous-time  UseExternalTs=off  SampleTime=-1  IntegratorMethod=Forward Euler  FilterMethod=Forward Euler  ControllerParametersSource=internal  P=Kpi_4DG  I=Kii_4DG  D=0  UseFilter=on  N=100  TunerSelectOption=Transfer Function Based (PID Tuner App)  InitialConditionSource=internal  InitialConditionForIntegrator=0  InitialConditionForFilter=0  DifferentiatorICPrevScaledInput=0  ExternalReset=none  TrackingMode=off  Kt=1  LimitOutput=off  SatLimitsSource=internal  UpperSaturationLimit=inf  LowerSaturationLimit=-inf  LinearizeAsGain=on  AntiWindupMode=none  Kb=1  POutMin=[]  POutMax=[]  IOutMin=[]  IOutMax=[]  DOutMin=[]  DOutMax=[]  NOutMin=[]  NOutMax=[]  SumOutMin=[]  SumOutMax=[]  SaturationOutMin=[]  SaturationOutMax=[]  PParamMin=[]  PParamMax=[]  IParamMin=[]  IParamMax=[]  DParamMin=[]  DParamMax=[]  NParamMin=[]  NParamMax=[]  KbParamMin=[]  KbParamMax=[]  KtParamMin=[]  KtParamMax=[]  KbOutMin=[]  KbOutMax=[]  KtOutMin=[]  KtOutMax=[]  IntegratorOutMin=[]  IntegratorOutMax=[]  FilterOutMin=[]  FilterOutMax=[]  SumI1OutMin=[]  SumI1OutMax=[]  SumI2OutMin=[]  SumI2OutMax=[]  SumI3OutMin=[]  SumI3OutMax=[]  SumI4OutMin=[]  SumI4OutMax=[]  SumDOutMin=[]  SumDOutMax=[]  DifferentiatorOutMin=[]  DifferentiatorOutMax=[]  FilterDiffOutCoefMin=[]  FilterDiffOutCoefMax=[]  ReciprocalOutMin=[]  ReciprocalOutMax=[]  SumDenOutMin=[]  SumDenOutMax=[]  SumNumOutMin=[]  SumNumOutMax=[]  DivideOutMin=[]  DivideOutMax=[]  UdiffTsProdOutMin=[]  UdiffTsProdOutMax=[]  NTsProdOutMin=[]  NTsProdOutMax=[]  UintegralTsProdOutMin=[]  UintegralTsProdOutMax=[]  UngainTsProdOutMin=[]  UngainTsProdOutMax=[]  IntegratorContinuousStateAttributes=''  IntegratorStateMustResolveToSignalObject=off  IntegratorRTWStateStorageClass=Auto  FilterContinuousStateAttributes=''  FilterStateMustResolveToSignalObject=off  FilterRTWStateStorageClass=Auto  ParallelPVariant=InternalParameters  IdealPVariant=Disabled  IVariant=InternalParameters  DVariant=Disabled  IntegratorVariant=Continuous  SatVariant=Disabled  AWVariant=Passthrough  PCopyVariant=Disabled  TRVariant=Disabled  FdbkBlocksVariant=Forward  IdealPFdbkVariant=Disabled  SatFdbkVariant=Disabled  DerivativeFilterVariant=Disabled  NVariant=Disabled  NCopyVariant=Disabled_SignalSpec  FilterICVariant=Disabled  IntegratorICVariant=InternalICs  ExternalResetVariant=Disabled  TRSumVariant=Passthrough  SumFdbkVariant=Disabled  SumVariant=Sum_PI  TsampFilterVariant=InternalTs  TsampNgainVariant=Passthrough  TsampIntegralVariant=Passthrough  ExternalSaturationOutDataTypeStr=Inherit: Same as second input
  PID Controller1 : pid_lib/PID Controller  Controller=PI  Form=Parallel  TimeDomain=Continuous-time  UseExternalTs=off  SampleTime=-1  IntegratorMethod=Forward Euler  FilterMethod=Forward Euler  ControllerParametersSource=internal  P=Kpi_4DG  I=Kii_4DG  D=0  UseFilter=on  N=100  TunerSelectOption=Transfer Function Based (PID Tuner App)  InitialConditionSource=internal  InitialConditionForIntegrator=0  InitialConditionForFilter=0  DifferentiatorICPrevScaledInput=0  ExternalReset=none  TrackingMode=off  Kt=1  LimitOutput=off  SatLimitsSource=internal  UpperSaturationLimit=inf  LowerSaturationLimit=-inf  LinearizeAsGain=on  AntiWindupMode=none  Kb=1  POutMin=[]  POutMax=[]  IOutMin=[]  IOutMax=[]  DOutMin=[]  DOutMax=[]  NOutMin=[]  NOutMax=[]  SumOutMin=[]  SumOutMax=[]  SaturationOutMin=[]  SaturationOutMax=[]  PParamMin=[]  PParamMax=[]  IParamMin=[]  IParamMax=[]  DParamMin=[]  DParamMax=[]  NParamMin=[]  NParamMax=[]  KbParamMin=[]  KbParamMax=[]  KtParamMin=[]  KtParamMax=[]  KbOutMin=[]  KbOutMax=[]  KtOutMin=[]  KtOutMax=[]  IntegratorOutMin=[]  IntegratorOutMax=[]  FilterOutMin=[]  FilterOutMax=[]  SumI1OutMin=[]  SumI1OutMax=[]  SumI2OutMin=[]  SumI2OutMax=[]  SumI3OutMin=[]  SumI3OutMax=[]  SumI4OutMin=[]  SumI4OutMax=[]  SumDOutMin=[]  SumDOutMax=[]  DifferentiatorOutMin=[]  DifferentiatorOutMax=[]  FilterDiffOutCoefMin=[]  FilterDiffOutCoefMax=[]  ReciprocalOutMin=[]  ReciprocalOutMax=[]  SumDenOutMin=[]  SumDenOutMax=[]  SumNumOutMin=[]  SumNumOutMax=[]  DivideOutMin=[]  DivideOutMax=[]  UdiffTsProdOutMin=[]  UdiffTsProdOutMax=[]  NTsProdOutMin=[]  NTsProdOutMax=[]  UintegralTsProdOutMin=[]  UintegralTsProdOutMax=[]  UngainTsProdOutMin=[]  UngainTsProdOutMax=[]  IntegratorContinuousStateAttributes=''  IntegratorStateMustResolveToSignalObject=off  IntegratorRTWStateStorageClass=Auto  FilterContinuousStateAttributes=''  FilterStateMustResolveToSignalObject=off  FilterRTWStateStorageClass=Auto  ParallelPVariant=InternalParameters  IdealPVariant=Disabled  IVariant=InternalParameters  DVariant=Disabled  IntegratorVariant=Continuous  SatVariant=Disabled  AWVariant=Passthrough  PCopyVariant=Disabled  TRVariant=Disabled  FdbkBlocksVariant=Forward  IdealPFdbkVariant=Disabled  SatFdbkVariant=Disabled  DerivativeFilterVariant=Disabled  NVariant=Disabled  NCopyVariant=Disabled_SignalSpec  FilterICVariant=Disabled  IntegratorICVariant=InternalICs  ExternalResetVariant=Disabled  TRSumVariant=Passthrough  SumFdbkVariant=Disabled  SumVariant=Sum_PI  TsampFilterVariant=InternalTs  TsampNgainVariant=Passthrough  TsampIntegralVariant=Passthrough  ExternalSaturationOutDataTypeStr=Inherit: Same as second input
  Product : Product
  Product1 : Product
  Selector1 : Selector  InputPortWidth=3  IndexOptions=Index vector (dialog)  Indices=[1 2]  OutputSizes=1
  Selector3 : Selector  InputPortWidth=3  IndexOptions=Index vector (dialog)  Indices=[1 2]  OutputSizes=1
  Sum : Sum  Inputs=|+-
  Sum1 : Sum  Inputs=|+-
  Sum2 : Sum  Inputs=|+-
  Sum3 : Sum  Inputs=|++
  powergui : powerlib/powergui  Priority=1  SimulationMode=Discrete  SampleTime=2e-6  frequency=60  Iterations=50  frequencyindice=0  Pbase=100e6  ErrMax=1e-4  UnitsV=kV  UnitsW=MW  buscounter=0  FunctionMessages=off  echomessages=off  EnableUseOfTLC=off  CurrentSourceSwitches=off  DisableSnubberDevices=off  DisableRonSwitches=off  DisableVfSwitches=off  DisplayEquations=off  AutomaticDiscreteSolvers=off  SolverType=Tustin/Backward Euler (TBE)  Interpol=off  ExternalGateDelay=off  methode=off  Ts=100  x0status=blocks  SPID=on  SwTol=0  HookPort=off  NonlinearTolerance=1e-4  nMaxIteration=100  ContinueOnMaxIteration=off  RestoreLinks=warning  ResistiveCurrentMeasurement=off  Frange=[0:2:500]  Ylog=off  Xlog=on  ShowGrid=off  save=off  variable=ZData  structure=0  ZoomFFT=off  StartTime=0.0  cycles=1  DisplayStyle=1  fundamental=60  FreqAxis=off  MaxFrequency=1000  frequencyindicesteady=1  RmsSteady=1  display=off
  v_s_ref_dq0_4DG : Outport
  wires:
  i_s_ref_dq0_4DG/1 -> Selector1/1
  Selector1/1 -> Demux/1
  i_s_dq0_4DG/1 -> Selector3/1
  Selector3/1 -> Demux2/1
  Demux/1 -> Sum/1
  Demux2/1 -> Product1/2, Sum/2
  Sum/1 -> PID Controller/1
  PID Controller/1 -> Sum1/1
  w_base_4DG/1 -> Gain/1
  Gain/1 -> Product1/1, Product/1
  Demux2/2 -> Product/2, Sum2/2
  Product/1 -> Sum1/2
  Demux/2 -> Sum2/1
  Sum2/1 -> PID Controller1/1
  PID Controller1/1 -> Sum3/1
  Product1/1 -> Sum3/2
  Mux/1 -> v_s_ref_dq0_4DG/1
  Sum1/1 -> Mux/1
  Sum3/1 -> Mux/2
  Constant/1 -> Mux/3

== system Grid_Forming_Converters_Microgrid_Github/DG 4 VCVSI /Primary Controller DG 4/Droop Control Subsystem 4 DG ==
  Q_4DG : Inport
  P_4DG : Inport  Port=2
  w_n_4DG : Inport  Port=3
  V_n_4DG : Inport  Port=4
  Constant : Constant  Value=0
  Gain : Gain  Gain=m_P_4DG
  Gain1 : Gain  Gain=n_Q_4DG
  Gain2 : Gain  Gain=1/(2*pi)
  Mux : Mux  Inputs=3
  Sum : Sum  Inputs=|+-
  Sum1 : Sum  Inputs=|+-
  powergui : powerlib/powergui  Priority=1  SimulationMode=Discrete  SampleTime=2e-6  frequency=60  Iterations=50  frequencyindice=0  Pbase=100e6  ErrMax=1e-4  UnitsV=kV  UnitsW=MW  buscounter=0  FunctionMessages=off  echomessages=off  EnableUseOfTLC=off  CurrentSourceSwitches=off  DisableSnubberDevices=off  DisableRonSwitches=off  DisableVfSwitches=off  DisplayEquations=off  AutomaticDiscreteSolvers=off  SolverType=Tustin/Backward Euler (TBE)  Interpol=off  ExternalGateDelay=off  methode=off  Ts=100  x0status=blocks  SPID=on  SwTol=0  HookPort=off  NonlinearTolerance=1e-4  nMaxIteration=100  ContinueOnMaxIteration=off  RestoreLinks=warning  ResistiveCurrentMeasurement=off  Frange=[0:2:500]  Ylog=off  Xlog=on  ShowGrid=off  save=off  variable=ZData  structure=0  ZoomFFT=off  StartTime=0.0  cycles=1  DisplayStyle=1  fundamental=60  FreqAxis=off  MaxFrequency=1000  frequencyindicesteady=1  RmsSteady=1  display=off
  w_4DG : Outport
  frequency_4DG : Outport  Port=2
  v_ref_dq0_4DG : Outport  Port=3
  wires:
  P_4DG/1 -> Gain/1
  Q_4DG/1 -> Gain1/1
  w_n_4DG/1 -> Sum/1
  Gain/1 -> Sum/2
  V_n_4DG/1 -> Sum1/1
  Gain1/1 -> Sum1/2
  Sum/1 -> Gain2/1, w_4DG/1
  Sum1/1 -> [v_odi_star_4DG], Mux/1
  Mux/1 -> v_ref_dq0_4DG/1
  Constant/1 -> [v_oq_star_4DG], Mux/3, Mux/2
  Gain2/1 -> frequency_4DG/1
